simulink model "CurrentSensor"  (R2022b)
settings: Solver=VariableStepAuto  StartTime=0.0  StopTime=6  RelTol=1e-3
libraries: dsparch4 x1
settings Model: Creator=mique  LastModifiedBy=ramuj
settings DataIOCC: ReturnWorkspaceOutputs=off

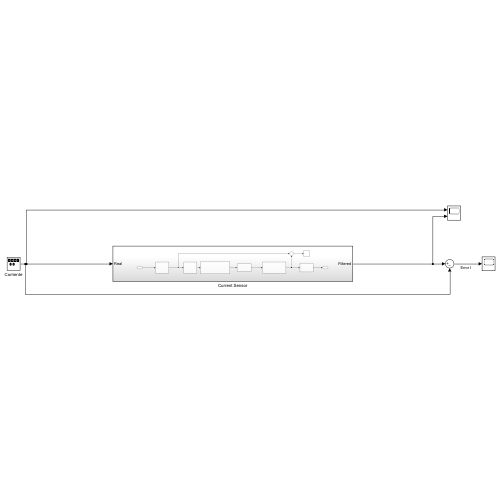
[thumbnail: Simulink's stored preview of the top-level diagram]
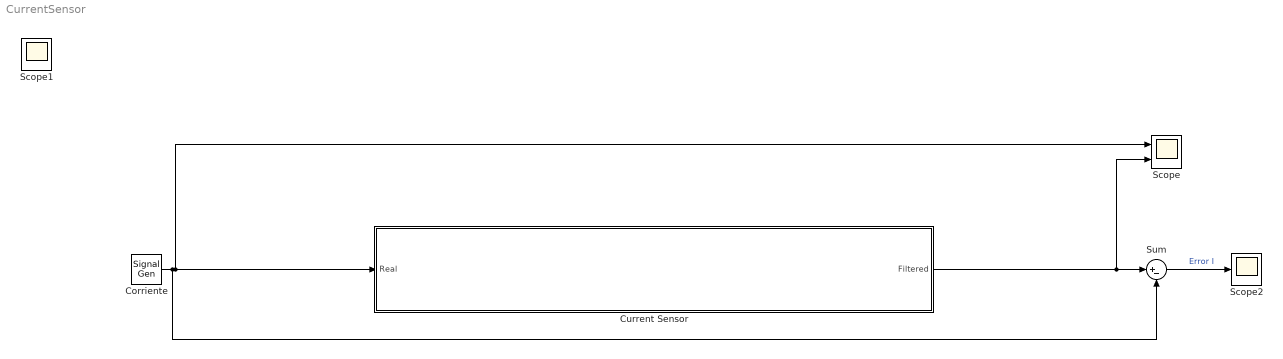
== system CurrentSensor ==
  Corriente : SignalGenerator  Amplitude=300
  Current Sensor : Subsystem
  Scope : Scope  NumInputPorts=2
  Scope2 : Scope
  Sum : Sum  Inputs=|+-
  Scope1 : Scope
  wires:
  Corriente/1 -> Sum/2, Scope/1, Current Sensor/1(Real)
  Sum/1 -> Scope2/1  "Error I"
  Current Sensor/1(Filtered) -> Scope/2, Sum/1

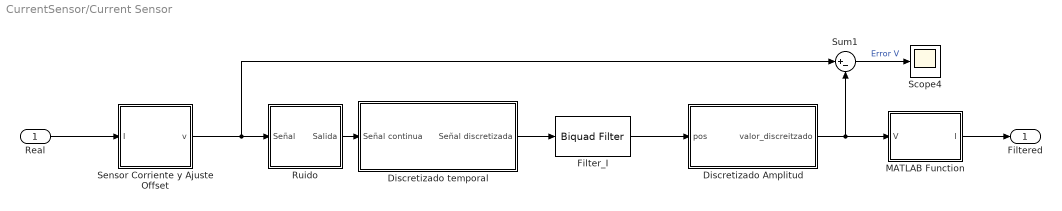
== system CurrentSensor/Current Sensor ==
  Real : Inport
  Discretizado Amplitud : Subsystem  mask{Num_Val=50, Max=4, Min=1}
      mask prompts: Num_Val "Numero de valores distintos"; Max "Maximo valor"; Min "Minimo valor"
  Discretizado temporal : Subsystem  mask{Tiempo_Discretizado=0.0001}
      mask prompts: Tiempo_Discretizado "Tiempo de discretizacion (s)"
      mask DialogControl DescGroupVar Prompt: Discretiza una señal mediante un ZOH con un tiempo definido
  Filter_I : dsparch4/Biquad Filter  Tag=BlockMethodSubSystem  FilterSource=Dialog parameters  CoeffSource=Specify via dialog  FilterObject=BQF  IIRFiltStruct=Direct form II  BiQuadCoeffs=[1 2 1 1 -1.7347257688092752 0.766006600943263893]  ScaleValues=[0.0078202080334971915;1]  IC=0  ICnum=0  ICden=0  a0Flag=Warning  optimizeScaleValues=on  ScaleValueMode=Specify via input port (g)  roundingMode=Floor  overflowMode=off  scaleValueFracLength=14  denProdOutputFracLength=30  denAccumFracLength=30  secondMemoryFracLength=15
  MATLAB Function : MATLAB Function  TreatAsAtomicUnit=on
  Ruido : Subsystem  mask{M=0, V=0.001, f=50}
      mask prompts: M "Media"; V "Varianza"; f "Frecuencia (Hz)"
      mask init:
      | T=1/f;
      mask DialogControl DescGroupVar Prompt: Añadidor de Ruido
      mask DialogControl DescTextVar Prompt: Añade un ruido blanco Gausiano con los siguientes valores:
  Scope4 : Scope
  Sensor Corriente y Ajuste Offset : Subsystem  mask{offset=0.003, max=off}
      mask prompts: max "Offset positivo"
      mask init:
      | if(max==true)
      |         offset=abs(offset);
      | 
      |     else
      |         offset=-offset;
      |     end
  Sum1 : Sum  Inputs=|+-
  Filtered : Outport
  wires:
  Sensor Corriente y Ajuste Offset/1(v) -> Ruido/1(Señal), Sum1/1
  Filter_I/1 -> Discretizado Amplitud/1(pos)
  Discretizado temporal/1(Señal discretizada) -> Filter_I/1
  Sum1/1 -> Scope4/1  "Error V"
  Discretizado Amplitud/1(valor_discreitzado) -> Sum1/2, MATLAB Function/1(V)
  Real/1 -> Sensor Corriente y Ajuste Offset/1(I)
  Ruido/1(Salida) -> Discretizado temporal/1(Señal continua)
  MATLAB Function/1(I) -> Filtered/1

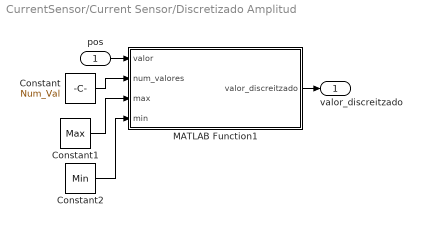
== system CurrentSensor/Current Sensor/Discretizado Amplitud ==
  pos : Inport
  Constant : Constant  Value=Num_Val
  Constant1 : Constant  Value=Max
  Constant2 : Constant  Value=Min
  MATLAB Function1 : MATLAB Function  TreatAsAtomicUnit=on
  valor_discreitzado : Outport
  wires:
  pos/1 -> MATLAB Function1/1(valor)
  Constant2/1 -> MATLAB Function1/4(min)
  Constant/1 -> MATLAB Function1/2(num_valores)
  Constant1/1 -> MATLAB Function1/3(max)
  MATLAB Function1/1(valor_discreitzado) -> valor_discreitzado/1

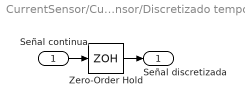
== system CurrentSensor/Current Sensor/Discretizado temporal ==
  Señal continua : Inport
  Zero-Order Hold : ZeroOrderHold  SampleTime=Tiempo_Discretizado
  Señal discretizada : Outport
  wires:
  Zero-Order Hold/1 -> Señal discretizada/1
  Señal continua/1 -> Zero-Order Hold/1

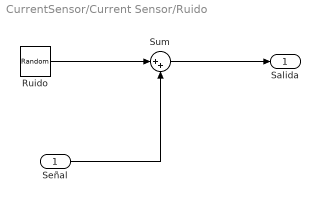
== system CurrentSensor/Current Sensor/Ruido ==
  Señal : Inport
  Ruido : RandomNumber  Mean=M  Variance=V  Seed=10  SampleTime=T
  Sum : Sum  Inputs=|++
  Salida : Outport
  wires:
  Sum/1 -> Salida/1
  Ruido/1 -> Sum/1
  Señal/1 -> Sum/2

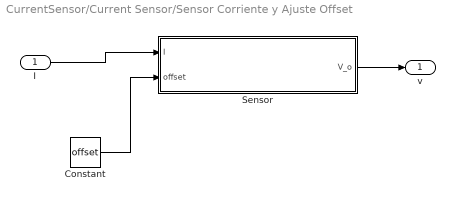
== system CurrentSensor/Current Sensor/Sensor Corriente y Ajuste Offset ==
  I : Inport
  Constant : Constant  Value=offset
  Sensor : MATLAB Function  TreatAsAtomicUnit=on
  v : Outport
  wires:
  I/1 -> Sensor/1(I)
  Constant/1 -> Sensor/2(offset)
  Sensor/1(V_o) -> v/1

== matlab function CurrentSensor/Current Sensor/Discretizado Amplitud/MATLAB Function1 ==
  data: valor input; valor_discreitzado output; num_valores input; max input; min input
function valor_discreitzado  = fcn(valor,num_valores,max,min)

if(valor>max)
    valor_discreitzado=max;
    return
end
if(valor<min)
    valor_discreitzado=min;
    return
end


valor_escalon=(max-min)/(num_valores-1);


i=min;
 while(i<max)
    if(i+valor_escalon/2>valor)
        valor_discreitzado=i;
        return
    end
    i=i+valor_escalon;
end



      valor_discreitzado=max;
end

== matlab function CurrentSensor/Current Sensor/Sensor Corriente y Ajuste Offset/Sensor ==
  data: I input; V_o output; offset input
function V_o = Sensor_L01Z300S05(I,offset)
Vcc=5;
if(I>300)
    I=300;
end
if(I<-300)
    I=-300;
end
V_ref=Vcc/2;
V_o=V_ref+0.005*I;

V_o=V_o+offset;

end

== matlab function CurrentSensor/Current Sensor/MATLAB Function ==
  data: V input; I output
function I = fcn(V)

I=(V-2.5)/0.005;
